simulink model "ssae1stpart"  (R2018b)
settings: Solver=VariableStepAuto  StartTime=0.0  StopTime=10.0  RelTol=1e-3
values from neighbouring files (symbols this model uses):
  A1 = [0 1;0 -1.9375]    [ssaelab2.m]
  B1 = [0;0.3125]    [ssaelab2.m]
  C1 = eye(2)    [ssaelab2.m]
  initial1 = [0.5 3]    [ssaelab2.m]
  KC = [KC1 KC2]    [ssaelab2.m]
  KC1 = 100    [ssaelab2.m]
  Pos = 0.3    [ssaelab2.m]
settings Model: Creator=user  LastModifiedBy=user

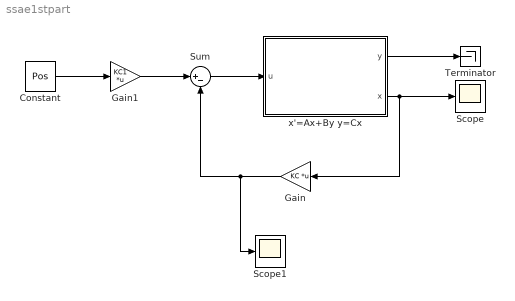
== system ssae1stpart ==
  Constant : Constant  Value=Pos
  Gain : Gain  Gain=KC  Multiplication=Matrix(K*u)
  Gain1 : Gain  Gain=KC1  Multiplication=Matrix(K*u)
  Scope : Scope
  Scope1 : Scope
  Sum : Sum  Inputs=|+-
  Terminator : Terminator
  x'=Ax+By y=Cx : Subsystem
  wires:
  x'=Ax+By y=Cx/1(y) -> Terminator/1
  Gain/1 -> Scope1/1, Sum/2
  Sum/1 -> x'=Ax+By y=Cx/1(u)
  x'=Ax+By y=Cx/2(x) -> Gain/1, Scope/1
  Constant/1 -> Gain1/1
  Gain1/1 -> Sum/1

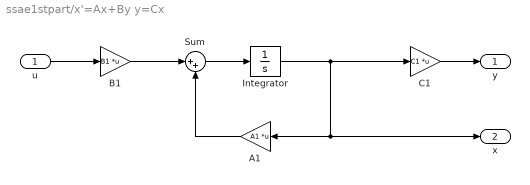
== system ssae1stpart/x'=Ax+By y=Cx ==
  u : Inport
  A1 : Gain  Gain=A1  Multiplication=Matrix(K*u)
  B1 : Gain  Gain=B1  Multiplication=Matrix(K*u)
  C1 : Gain  Gain=C1  Multiplication=Matrix(K*u)
  Integrator : Integrator  InitialCondition=initial1
  Sum : Sum  Inputs=|++
  y : Outport
  x : Outport  Port=2
  wires:
  A1/1 -> Sum/2
  u/1 -> B1/1
  Integrator/1 -> C1/1, x/1, A1/1
  B1/1 -> Sum/1
  Sum/1 -> Integrator/1
  C1/1 -> y/1
